simulink model "TransformationDerivationTest"  (R2019b)
settings: Solver=VariableStepAuto  StartTime=0.0  StopTime=10.0  RelTol=1e-3
libraries: roblocks x11
settings Model: Creator=Karl  LastModifiedBy=Karl

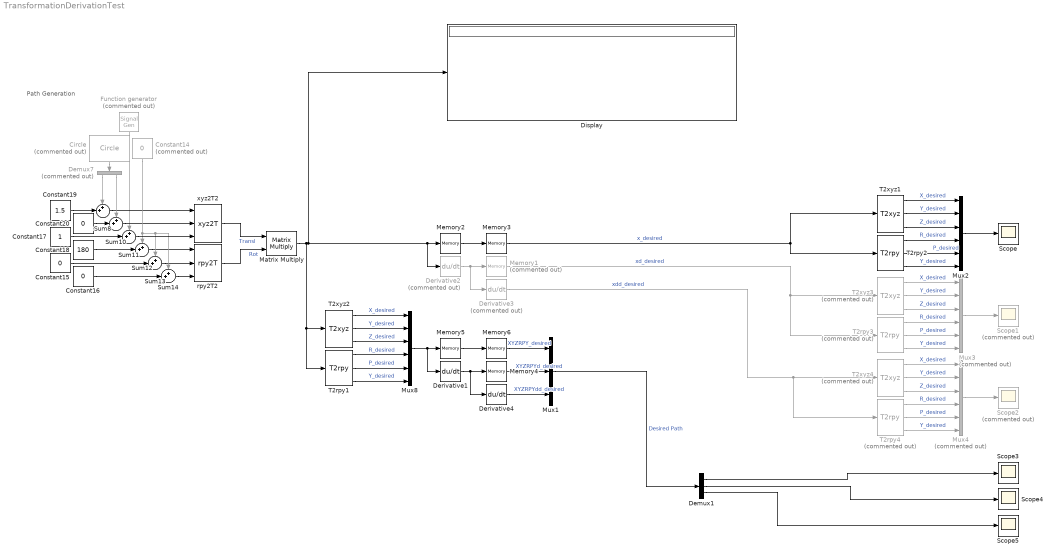
== system TransformationDerivationTest ==
  note: Path Generation
  "Circle " : roblocks/Toolbox/Circle  Commented=on  radius=0.5  freq=0.1
  Constant14 : Constant  Commented=on  Value=0
  Constant15 : Constant  Value=0
  Constant16 : Constant  Value=0
  Constant17 : Constant
  Constant18 : Constant  Value=180
  Constant19 : Constant  Value=1.5
  Constant20 : Constant  Value=0
  Demux1 : Demux  Outputs=3
  Demux7 : Demux  Commented=on  Outputs=2
  Derivative1 : Derivative
  Derivative2 : Derivative  Commented=on
  Derivative3 : Derivative  Commented=on
  Derivative4 : Derivative
  Display : Display
  Function generator : SignalGenerator  Commented=on  Amplitude=0.2
  Matrix Multiply : Product  Multiplication=Matrix(*)
  Memory1 : Memory  Commented=on  InitialCondition=ones(4)  InheritSampleTime=on
  Memory2 : Memory  InitialCondition=ones(4)  InheritSampleTime=on
  Memory3 : Memory  InitialCondition=ones(4)  InheritSampleTime=on
  Memory4 : Memory  InitialCondition=[0 0 0 0 0 0]  InheritSampleTime=on
  Memory5 : Memory  InitialCondition=[0 0 0 0 0 0]  InheritSampleTime=on
  Memory6 : Memory  InitialCondition=[0 0 0 0 0 0]  InheritSampleTime=on
  Mux1 : Mux  Inputs=3
  Mux2 : Mux  Inputs=6
  Mux3 : Mux  Commented=on  Inputs=6
  Mux4 : Mux  Commented=on  Inputs=6
  Mux8 : Mux  Inputs=6
  Scope{,3..5} (4 alike) : Scope
  Scope1 : Scope  Commented=on
  Scope2 : Scope  Commented=on
  Sum{8,10..14} (6 alike) : Sum  Inputs=++|
  T2rpy1 : roblocks/Toolbox/T2rpy  sequence=ZYX  degrees=off
  T2rpy2 : roblocks/Toolbox/T2rpy  sequence=ZYX  degrees=off
  T2rpy3 : roblocks/Toolbox/T2rpy  Commented=on  sequence=ZYX  degrees=off
  T2rpy4 : roblocks/Toolbox/T2rpy  Commented=on  sequence=ZYX  degrees=off
  T2xyz1 : roblocks/Toolbox/T2xyz
  T2xyz2 : roblocks/Toolbox/T2xyz
  T2xyz3 : roblocks/Toolbox/T2xyz  Commented=on
  T2xyz4 : roblocks/Toolbox/T2xyz  Commented=on
  rpy2T2 : roblocks/Toolbox/rpy2T  sequence=ZYX  degrees=on
  xyz2T2 : roblocks/Toolbox/xyz2T
  wires:
  T2rpy1/2 -> Mux8/5  "P_desired"
  T2xyz2/3 -> Mux8/3  "Z_desired"
  T2xyz2/2 -> Mux8/2  "Y_desired"
  Sum13/1 -> rpy2T2/2
  "Circle "/1 -> Demux7/1
  Derivative2/1 -> Memory1/1, Derivative3/1
  Function generator/1 -> Sum11/1
  Sum10/1 -> xyz2T2/2
  Sum8/1 -> xyz2T2/1
  Sum12/1 -> rpy2T2/1
  Constant18/1 -> Sum12/2
  Demux7/2 -> Sum10/1
  Constant15/1 -> Sum13/2
  Constant19/1 -> Sum8/2
  Constant16/1 -> Sum14/2
  Memory1/1 -> T2rpy3/1, T2xyz3/1  "xd_desired"
  Derivative3/1 -> T2rpy4/1, T2xyz4/1  "xdd_desired"
  Constant14/1 -> Sum14/1, Sum13/1, Sum12/1
  Sum14/1 -> rpy2T2/3
  Constant20/1 -> Sum10/2
  Sum11/1 -> xyz2T2/3
  Memory2/1 -> Memory3/1
  T2rpy1/1 -> Mux8/4  "R_desired"
  Memory3/1 -> T2rpy2/1, T2xyz1/1  "x_desired"
  T2rpy1/3 -> Mux8/6  "Y_desired"
  Demux7/1 -> Sum8/1
  xyz2T2/1 -> Matrix Multiply/1  "Transl"
  T2xyz2/1 -> Mux8/1  "X_desired"
  Constant17/1 -> Sum11/2
  Matrix Multiply/1 -> T2rpy1/1, T2xyz2/1, Display/1, Memory2/1, Derivative2/1
  rpy2T2/1 -> Matrix Multiply/2  "Rot"
  Derivative1/1 -> Memory4/1, Derivative4/1
  Derivative4/1 -> Mux1/3  "XYZRPYdd_desired"
  Mux8/1 -> Derivative1/1, Memory5/1
  Memory4/1 -> Mux1/2  "XYZRPYd_desired"
  Memory5/1 -> Memory6/1
  Memory6/1 -> Mux1/1  "XYZRPY_desired"
  T2xyz1/2 -> Mux2/2  "Y_desired"
  T2rpy2/2 -> Mux2/5  "P_desired"
  T2xyz1/3 -> Mux2/3  "Z_desired"
  T2rpy2/3 -> Mux2/6  "Y_desired"
  T2rpy2/1 -> Mux2/4  "R_desired"
  T2xyz1/1 -> Mux2/1  "X_desired"
  T2rpy3/1 -> Mux3/4  "R_desired"
  T2rpy3/3 -> Mux3/6  "Y_desired"
  T2xyz3/3 -> Mux3/3  "Z_desired"
  T2rpy3/2 -> Mux3/5  "P_desired"
  T2xyz3/1 -> Mux3/1  "X_desired"
  T2xyz3/2 -> Mux3/2  "Y_desired"
  T2rpy4/1 -> Mux4/4  "R_desired"
  T2rpy4/3 -> Mux4/6  "Y_desired"
  T2xyz4/3 -> Mux4/3  "Z_desired"
  T2rpy4/2 -> Mux4/5  "P_desired"
  T2xyz4/1 -> Mux4/1  "X_desired"
  T2xyz4/2 -> Mux4/2  "Y_desired"
  Mux1/1 -> Demux1/1  "Desired Path"
  Mux2/1 -> Scope/1
  Mux3/1 -> Scope1/1
  Mux4/1 -> Scope2/1
  Demux1/1 -> Scope3/1
  Demux1/2 -> Scope4/1
  Demux1/3 -> Scope5/1
